simulink subsystem "ABS_simulink_20a"  (R2020a)
settings: Solver=VariableStepAuto  StartTime=0.0  StopTime=10.0  RelTol=1e-3
settings Model: Creator=126893  LastModifiedBy=126893
settings DebuggingCC: UnconnectedInputMsg=none  UnconnectedOutputMsg=none  UnconnectedLineMsg=none  SFMachineParentedDataDiag=error
settings ModelReferenceCC: EnableRefExpFcnMdlSchedulingChecks=off
settings RTWCC: Description=Generic Real-Time Target

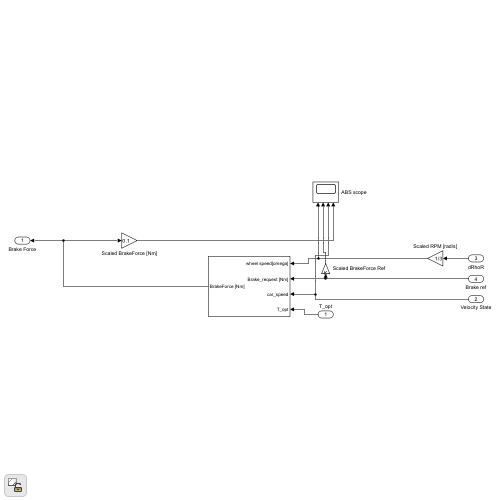
[thumbnail: Simulink's stored preview of the top-level diagram]
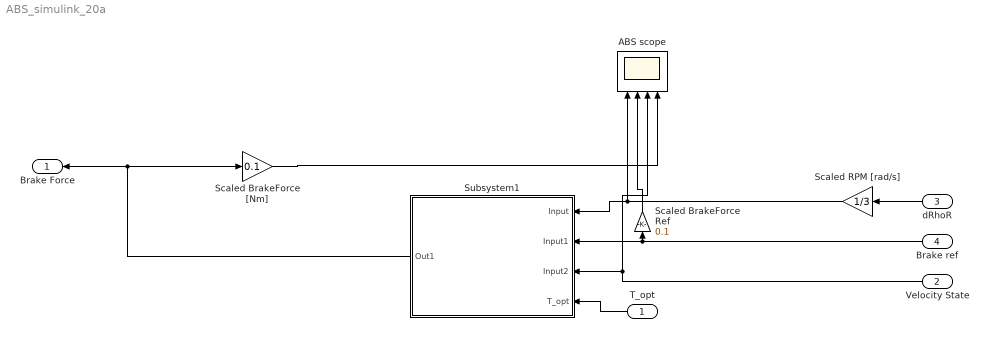
== system ABS_simulink_20a ==
  T_opt : Inport
  Velocity State : Inport  Port=2
  dRhoR : Inport  Port=3
  Brake ref : Inport  Port=4
  ABS scope : Scope  NumInputPorts=4
  Scaled BrakeForce Ref : Gain  Gain=0.1
  Scaled BrakeForce [Nm] : Gain  Gain=0.1
  Scaled RPM [rad/s] : Gain  Gain=1/3
  Subsystem1 : Subsystem
  Brake Force : Outport
  wires:
  Scaled BrakeForce [Nm]/1 -> ABS scope/4
  Scaled BrakeForce Ref/1 -> ABS scope/2
  Brake ref/1 -> Subsystem1/2(Input1), Scaled BrakeForce Ref/1
  Subsystem1/1(Out1) -> Brake Force/1, Scaled BrakeForce [Nm]/1
  Velocity State/1 -> ABS scope/3, Subsystem1/3(Input2)
  dRhoR/1 -> Scaled RPM [rad/s]/1
  Scaled RPM [rad/s]/1 -> ABS scope/1, Subsystem1/1(Input)
  T_opt/1 -> Subsystem1/4(T_opt)

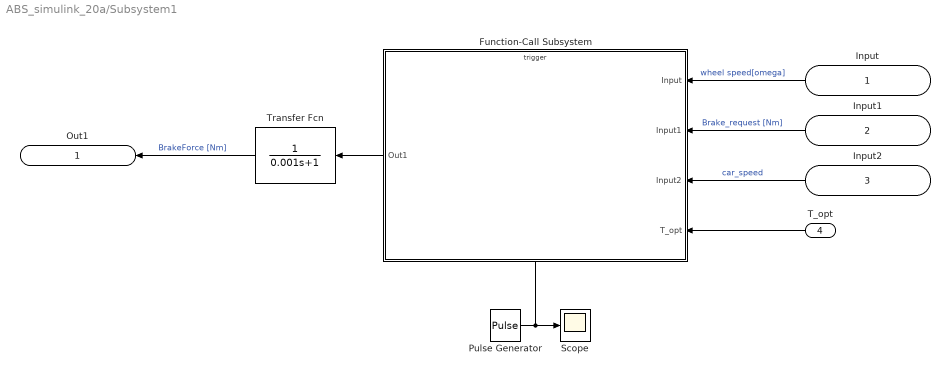
== system ABS_simulink_20a/Subsystem1 ==
  Input : Inport
  Input1 : Inport  Port=2
  Input2 : Inport  Port=3
  T_opt : Inport  Port=4
  Function-Call Subsystem : Subsystem  TreatAsAtomicUnit=on
  Pulse Generator : DiscretePulseGenerator  PulseType=Time based  Period=0.001  PulseWidth=50
  Scope : Scope
  Transfer Fcn : TransferFcn  Denominator=[0.001 1]
  Out1 : Outport
  wires:
  T_opt/1 -> Function-Call Subsystem/4(T_opt)
  Pulse Generator/1 -> Function-Call Subsystem/Trigger, Scope/1
  Transfer Fcn/1 -> Out1/1  "BrakeForce [Nm]"
  Input2/1 -> Function-Call Subsystem/3(Input2)  "car_speed"
  Input1/1 -> Function-Call Subsystem/2(Input1)  "Brake_request [Nm]"
  Input/1 -> Function-Call Subsystem/1(Input)  "wheel speed[omega]"
  Function-Call Subsystem/1(Out1) -> Transfer Fcn/1

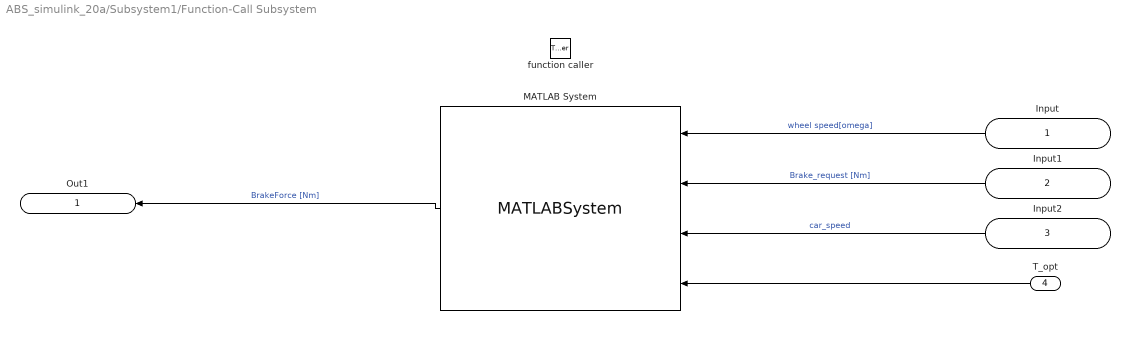
== system ABS_simulink_20a/Subsystem1/Function-Call Subsystem ==
  Input : Inport
  Input1 : Inport  Port=2
  Input2 : Inport  Port=3
  T_opt : Inport  Port=4
  function caller : TriggerPort  VariantControl=Variant
  MATLAB System : MATLABSystem  System=ABS  lambda_max=0  lambda_min_relaxing=0  lambda_min=0  fast_ramp=0  slow_ramp=0  fast_to_slow_slope_threshold=0  SimulateUsing=Code generation
      mask Type: ABS
      mask Display:
      | disp('ABS');
      | port_label('input',1,'rpm');
      | port_label('input',2,'max_brake');
      | port_label('input',3,'car_speed');
      | port_label('input',4,'T_opt');
      | port_label('output',1,'brake');
  Out1 : Outport
  wires:
  T_opt/1 -> MATLAB System/4
  Input2/1 -> MATLAB System/3  "car_speed"
  Input1/1 -> MATLAB System/2  "Brake_request [Nm]"
  Input/1 -> MATLAB System/1  "wheel speed[omega]"
  MATLAB System/1 -> Out1/1  "BrakeForce [Nm]"
